simulink model "NEXTCAR_Interface"  (R2017a)
settings: Solver=ode4  StartTime=0.0  StopTime=10000  FixedStep=0.001  RelTol=1e-3  EnableMultiTasking=on
undefined symbols (not defined in the file or in its folder): IO306
libraries: NEXTCAR_Library x50, speedgoatlib_IO106 x4, slrtlib x3, simulink x3, speedgoatlib_fpga_pwm x2, speedgoatlib_IO204 x2, slrttcplib x2, simulink_extras x2, speedgoatlib_fpga x1, xpcseriallib x1, powerlib_meascontrol x1
(part 1 of 2)
settings Model: sg_rtwmakecfg_data=_sglibc_  Creator=G Shaver TC2  LastModifiedBy=joreADM
settings SolverCC: EnableConcurrentExecution=on
settings DataIOCC: SaveFormat=Array  SaveState=on
settings OptimizationCC: BlockReduction=off  OptimizeBlockIOStorage=off  BufferReuse=off  GlobalBufferReuse=off  ExpressionFolding=off  LocalBlockOutputs=off  LifeSpan=inf
settings DebuggingCC: UnderspecifiedInitializationDetection=Classic  MergeDetectMultiDrivingBlocksExec=none  CheckExecutionContextRuntimeOutputMsg=on  SignalResolutionControl=TryResolveAllWithWarning  MultiTaskDSMMsg=warning  MultiTaskCondExecSysMsg=none  SFUnexpectedBacktrackingDiag=warning  SFNoUnconditionalDefaultTransitionDiag=warning
settings HardwareCC: ProdBitPerPointer=32  ProdBitPerSizeT=32  ProdBitPerPtrDiffT=32  ProdLargestAtomicFloat=None  ProdWordSize=32  ProdLongLongMode=on  ProdHWDeviceType=Generic->32-bit x86 compatible
settings RTWCC: SystemTargetFile=slrt.tlc  TemplateMakefile=slrt_default_tmf  Description=Simulink Real-Time  RTWCompilerOptimization=on
settings SimulinkRealTimeCC: xPCisDownloadable=off  xPCisModelTimeout=off  xPCModelTimeoutSecs=30
settings ConfigComp: CovMetricSettings=dw  CovHtmlReporting=on  CovSaveCumulativeToWorkspaceVar=on  CovSaveSingleToWorkspaceVar=on

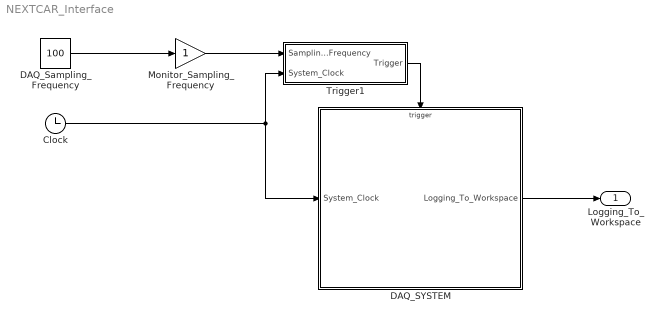
== system NEXTCAR_Interface ==
  Clock : Clock
  DAQ_SYSTEM : Subsystem
  DAQ_Sampling_Frequency : Constant  Value=100
  Monitor_Sampling_Frequency : Gain
  Trigger1 : Subsystem
  Logging_To_Workspace : Outport
  wires:
  Trigger1/1(Trigger) -> DAQ_SYSTEM/Trigger
  DAQ_SYSTEM/1(Logging_To_Workspace) -> Logging_To_Workspace/1
  DAQ_Sampling_Frequency/1 -> Monitor_Sampling_Frequency/1
  Clock/1 -> DAQ_SYSTEM/1(System_Clock), Trigger1/2(System_Clock)
  Monitor_Sampling_Frequency/1 -> Trigger1/1(Sampling_Frequency)

== system NEXTCAR_Interface/DAQ_SYSTEM ==
  note: DEBUG MODE
  System_Clock : Inport
  Trigger1 : TriggerPort  VariantControl=Variant
  Analog_IO_Interface : Subsystem
  Debug_Mode : Constant  Value=0
  Digital_IO_Interface : Subsystem
  Ethernet_Interface : Subsystem  TreatAsAtomicUnit=on
  Logging_Interface : Subsystem
  Mux : Mux
  System_Processing : Subsystem
  Trigger : Subsystem
  Trigger2 : Subsystem
  Logging_To_Workspace : Outport
  tag scope: Debug_Mode=global
  wires:
  Mux/1 -> Logging_Interface/1(Logging_Data), Logging_To_Workspace/1
  Trigger/1(Trigger) -> Ethernet_Interface/Trigger
  Debug_Mode/1 -> [Debug_Mode]
  System_Clock/1 -> Trigger2/1(System_Clock), Trigger/1(System_Clock)
  Trigger2/1(Trigger) -> Logging_Interface/2(Clock_Trigger)
  Analog_IO_Interface/1(Signal_Logging) -> Mux/1
  System_Processing/1(Signal_Logging) -> Mux/4
  Ethernet_Interface/1(Signal_Logging) -> Mux/3
  Digital_IO_Interface/1(Signal_Logging) -> Mux/2

== system NEXTCAR_Interface/Trigger1 ==
  Sampling_Frequency : Inport
  System_Clock : Inport  Port=2
  Constant : Constant
  Divide : Product  Inputs=*/
  Divide1 : Product  Inputs=*/
  Floor : Rounding
  Memory : Memory  InheritSampleTime=on
  Relational Operator : RelationalOperator  Operator=>  OutDataTypeStr=boolean  RndMeth=Simplest
  Trigger : Outport
  wires:
  System_Clock/1 -> Divide/1
  Relational Operator/1 -> Trigger/1
  Divide/1 -> Floor/1
  Memory/1 -> Relational Operator/2
  Floor/1 -> Memory/1, Relational Operator/1
  Sampling_Frequency/1 -> Divide1/2
  Divide1/1 -> Divide/2
  Constant/1 -> Divide1/1

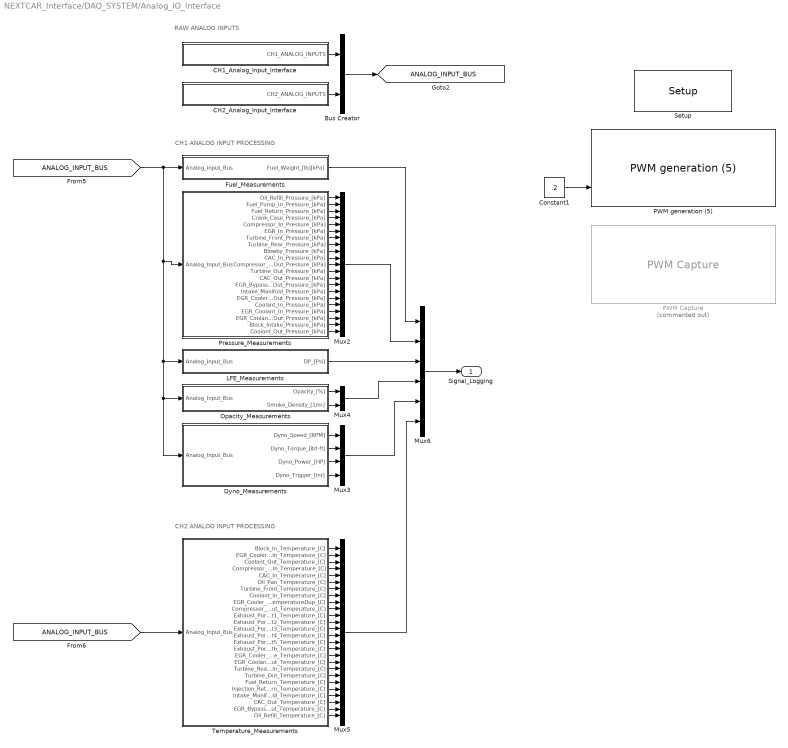
== system NEXTCAR_Interface/DAQ_SYSTEM/Analog_IO_Interface ==
  note: CH2 ANALOG INPUT PROCESSING
  note: CH1 ANALOG INPUT PROCESSING
  note: RAW ANALOG INPUTS
  Bus Creator : BusCreator  Inputs=2
  CH1_Analog_Input_Interface : Subsystem
  CH2_Analog_Input_Interface : Subsystem
  Constant1 : Constant  Value=.2
  Dyno_Measurements : Subsystem
  Fuel_Measurements : Subsystem
  LFE_Measurements : Subsystem
  Mux2 : Mux  Inputs=21
  Mux3 : Mux
  Mux4 : Mux  Inputs=2
  Mux5 : Mux  Inputs=26
  Mux6 : Mux  Inputs=6
  Opacity_Measurements : Subsystem
  PWM Capture : speedgoatlib_fpga_pwm/PWM Capture  Commented=on  id=1  chan=[1]  ts=0.001  pciSlot=-1  board=IO306-25k  captureMode=High transitions triggered  captureTimeout=0  showHighDuration=on  showLowDuration=on  showPeriod=on  showDC16=off  showDC8=off  showTOn=off  showTOff=off  showValidData=off
      settings: SourceProductName=Simulink Real-Time: Speedgoat I/O Driver Library
  PWM generation (5) : speedgoatlib_fpga_pwm/PWM generation (5)  id=1  chan=[1]  board=IO306-25k  ts=-1  pciSlot=-1  symmetric=Symmetric - PWM generation is centered around half the period  b_is_complement_of_a=Independent of PWM A output  deadband=[0.0]  period=0.001  frequency=1000  ticks=32999  a_on=[0]  a_off=[0]  pwm_a_dc=[0.0]  b_on=[0]  b_off=[0]  pwm_b_dc=[0]  c_on=[0.0]  c_off=[0.0]  protection=Disabled: A and B can be high at the same moment  enable_latch_half_period=off  trigger_duration=[1e-6]  trigger_period_start=off  trigger_half_of_the_period=off  trigger_a_on=off  trigger_a_off=off  trigger_b_on=off  trigger_b_off=off  show_a_input=on  show_b_input=on  show_c_input=off  show_period_input=off  show_force_stop_input=off  idle_a=Low when PWM generation is halted  idle_b=Low when PWM generation is halted  idle_c=Low when PWM generation is halted  cancels_pwm_generation=on  invert_a=off  invert_b=off  invert_c=off
      settings: SourceProductName=Simulink Real-Time: Speedgoat I/O Driver Library
  Pressure_Measurements : Subsystem
  Setup : speedgoatlib_fpga/Setup/Setup  board=IO306-25k  id=1  frontIO=None  rearIO=None  bitstreamFile=speedgoat_IO306_25k_CI_01697  timestamp_string=00/00/00 00:00:00  ProgSpiFlash=off  ProgBPIFlash=off  pciSlot=-1  PullRPort0=pull-up 3.3V  VioPort0=3.3V  PullRPort1=pull-up 3.3V  VioPort1=3.3V  PullRPort2=pull-up 3.3V  VioPort2=3.3V  PullRPort3=pull-up 3.3V  VioPort3=3.3V  PullRPort4=pull-up 3.3V  VioPort4=3.3V  PullRPort5=pull-up 3.3V  VioPort5=3.3V  PullRPort6=pull-up 3.3V  VioPort6=3.3V  PullRPort15=pull-up 3.3V  PullRPort31=pull-up 3.3V  PullRPort47=pull-up 3.3V  PullRPort63=pull-up 3.3V
      settings: SourceProductName=Simulink Real-Time: Speedgoat I/O Driver Library
  Temperature_Measurements : Subsystem
  Signal_Logging : Outport
  tag scope: ANALOG_INPUT_BUS=global
  wires:
  Mux6/1 -> Signal_Logging/1
  CH1_Analog_Input_Interface/1(CH1_ANALOG_INPUTS) -> Bus Creator/1
  [ANALOG_INPUT_BUS] -> Dyno_Measurements/1(Analog_Input_Bus), Opacity_Measurements/1(Analog_Input_Bus), LFE_Measurements/1(Analog_Input_Bus), Pressure_Measurements/1(Analog_Input_Bus), Fuel_Measurements/1("Analog_Input_Bus ")
  Dyno_Measurements/1(Dyno_Speed_[RPM]) -> Mux3/1
  Dyno_Measurements/2(Dyno_Torque_[lbf-ft]) -> Mux3/2
  Dyno_Measurements/3(Dyno_Power_[HP]) -> Mux3/3
  Dyno_Measurements/4(Dyno_Trigger_[int]) -> Mux3/4
  Opacity_Measurements/1(Opacity_[%]) -> Mux4/1
  Opacity_Measurements/2(Smoke_Density_[1/m]) -> Mux4/2
  [ANALOG_INPUT_BUS] -> Temperature_Measurements/1(Analog_Input_Bus)
  CH2_Analog_Input_Interface/1(CH2_ANALOG_INPUTS) -> Bus Creator/2
  Bus Creator/1 -> [ANALOG_INPUT_BUS]
  Pressure_Measurements/1(Oil_Refill_Pressure_[kPa]) -> Mux2/1
  Pressure_Measurements/2(Fuel_Pump_In_Pressure_[kPa]) -> Mux2/2
  Pressure_Measurements/3(Fuel_Return_Pressure_[kPa]) -> Mux2/3
  Pressure_Measurements/4(Crank_Case_Pressure_[kPa]) -> Mux2/4
  Pressure_Measurements/5(Compressor_In_Pressure_[kPa]) -> Mux2/5
  Pressure_Measurements/6(EGR_In_Pressure_[kPa]) -> Mux2/6
  Pressure_Measurements/7(Turbine_Front_Pressure_[kPa]) -> Mux2/7
  Pressure_Measurements/8(Turbine_Rear_Pressure_[kPa]) -> Mux2/8
  Pressure_Measurements/9(Blowby_Pressure_[kPa]) -> Mux2/9
  Pressure_Measurements/10(CAC_In_Pressure_[kPa]) -> Mux2/10
  Pressure_Measurements/11(Compressor_Out_Pressure_[kPa]) -> Mux2/11
  Pressure_Measurements/12(Turbine_Out_Pressure_[kPa]) -> Mux2/12
  Pressure_Measurements/13(CAC_Out_Pressure_[kPa]) -> Mux2/13
  Pressure_Measurements/14(EGR_Bypass_Out_Pressure_[kPa]) -> Mux2/14
  Pressure_Measurements/15(Intake_Manifold_Pressure_[kPa]) -> Mux2/15
  Pressure_Measurements/16(EGR_Cooler_Out_Pressure_[kPa]) -> Mux2/16
  Pressure_Measurements/17(Coolant_In_Pressure_[kPa]) -> Mux2/17
  Pressure_Measurements/18(EGR_Coolant_In_Pressure_[kPa]) -> Mux2/18
  Pressure_Measurements/19(EGR_Coolant_Out_Pressure_[kPa]) -> Mux2/19
  Pressure_Measurements/20(Block_Intake_Pressure_[kPa]) -> Mux2/20
  Pressure_Measurements/21(Coolant_Out_Pressure_[kPa]) -> Mux2/21
  Constant1/1 -> PWM generation (5)/2
  Temperature_Measurements/1(Block_In_Temperature_[C]) -> Mux5/1
  Temperature_Measurements/2(EGR_Cooler_In_Temperature_[C]) -> Mux5/2
  Temperature_Measurements/3(Coolant_Out_Temperature_[C]) -> Mux5/3
  Temperature_Measurements/4(Compressor_In_Temperature_[C]) -> Mux5/4
  Temperature_Measurements/5(CAC_In_Temperature_[C]) -> Mux5/5
  Temperature_Measurements/6(Oil_Pan_Temperature_[C]) -> Mux5/6
  Temperature_Measurements/7(Turbine_Front_Temperature_[C]) -> Mux5/7
  Temperature_Measurements/8(Coolant_In_Temperature_[C]) -> Mux5/8
  Temperature_Measurements/9(EGR_Cooler_In_TemperatureDup_[C]) -> Mux5/9
  Temperature_Measurements/10(Compressor_Out_Temperature_[C]) -> Mux5/10
  Temperature_Measurements/11(Exhaust_Port1_Temperature_[C]) -> Mux5/11
  Temperature_Measurements/12(Exhaust_Port2_Temperature_[C]) -> Mux5/12
  Temperature_Measurements/13(Exhaust_Port3_Temperature_[C]) -> Mux5/13
  Temperature_Measurements/14(Exhaust_Port4_Temperature_[C]) -> Mux5/14
  Temperature_Measurements/15(Exhaust_Port5_Temperature_[C]) -> Mux5/15
  Temperature_Measurements/16(Exhaust_Port6_Temperature_[C]) -> Mux5/16
  Temperature_Measurements/17(EGR_Cooler_Intake_Temperature_[C]) -> Mux5/17
  Temperature_Measurements/18(EGR_Coolant_Out_Temperature_[C]) -> Mux5/18
  Temperature_Measurements/19(Turbine_Rear_In_Temperature_[C]) -> Mux5/19
  Temperature_Measurements/20(Turbine_Out_Temperature_[C]) -> Mux5/20
  Temperature_Measurements/21(Fuel_Return_Temperature_[C]) -> Mux5/21
  Temperature_Measurements/22(Injection_Return_Temperature_[C]) -> Mux5/22
  Temperature_Measurements/23(Intake_Manifold_Temperature_[C]) -> Mux5/23
  Temperature_Measurements/24(CAC_Out_Temperature_[C]) -> Mux5/24
  Temperature_Measurements/25(EGR_Bypass_Out_Temperature_[C]) -> Mux5/25
  Temperature_Measurements/26(Oil_Refill_Temperature_[C]) -> Mux5/26
  Fuel_Measurements/1(Fuel_Weight_[lb][kPa]) -> Mux6/1
  Mux2/1 -> Mux6/2
  LFE_Measurements/1(DP_[Psi]) -> Mux6/3
  Mux4/1 -> Mux6/4
  Mux3/1 -> Mux6/5
  Mux5/1 -> Mux6/6

== system NEXTCAR_Interface/DAQ_SYSTEM/Digital_IO_Interface ==
  note: COMMANDED DIGITAL OUTPUTS
  Digital_Output_Interface : Subsystem
  Signal_Logging : Outport
  wires:
  Digital_Output_Interface/1(Signal_Logging) -> Signal_Logging/1

== system NEXTCAR_Interface/DAQ_SYSTEM/Ethernet_Interface ==
  Trigger : TriggerPort  VariantControl=Variant
  ASCII_Encode : xpcseriallib/ASCII Encode   format=%d  nvars=1  maxlength=3  vartypes={ 'double' }
      settings: SourceProductName=Simulink Real-Time  SourceProductBaseCode=XP
  Constant : Constant  Value=100
  Constant1 : Constant
  Mux : Mux  Inputs=2
  TCP_Client_Configure : slrttcplib/TCP Client Configure  Priority=-1  useHostTargetConn=off  clientAddress=192.168.7.2  clientPort=65001  SubnetMask=255.255.255.2  Gateway=0.0.0.0  remoteAddress=192.168.7.222  remotePort=10006  PciBus=7  PciSlot=6
      settings: SourceProductName=Simulink Real-Time  SourceProductBaseCode=XP
  TCP_Send : slrttcplib/TCP Send  socketAddPortVal=Client: 192.168.7.2:65001  sampleTime=-1
      settings: SourceProductName=Simulink Real-Time  SourceProductBaseCode=XP
  Width1 : Width
  Signal_Logging : Outport
  wires:
  Constant/1 -> ASCII_Encode/1
  Width1/1 -> TCP_Send/3
  ASCII_Encode/1 -> TCP_Send/2, Width1/1
  Constant1/1 -> TCP_Send/1, TCP_Client_Configure/1
  TCP_Client_Configure/1 -> Mux/1  "TCP_Client_Configure_Status_[-]"
  TCP_Send/1 -> Mux/2  "TCP_Send_Status_[-]"
  Mux/1 -> Signal_Logging/1

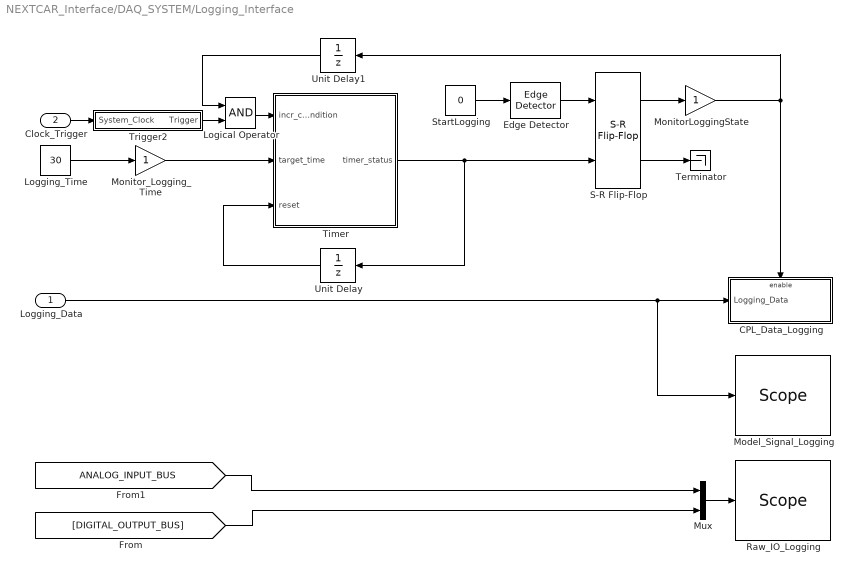
== system NEXTCAR_Interface/DAQ_SYSTEM/Logging_Interface ==
  Logging_Data : Inport
  Clock_Trigger : Inport  Port=2
  CPL_Data_Logging : Subsystem  TreatAsAtomicUnit=on
  Edge Detector : powerlib_meascontrol/Logic/Edge Detector  model=Either  ic=0  Ts=-1
      settings: SourceProductName=Simscape Power Systems  SourceProductBaseCode=PS
  Logging_Time : Constant  Value=30
  Logical Operator : Logic  AllPortsSameDT=off  OutDataTypeStr=boolean
  "Model_Signal_Logging " : slrtlib/Displays and Logging/Scope   scopeno=1  scopetype=File  autostart=on  viewmode=Graphical redraw  formatstr='%15.6f'  grid=on  ylimits=[0,0]  nosamples=250  noprepostsamples=0  interleave=1  triggermode=FreeRun  triggersignal=1  trigsignalfromport=on  triggerlevel=0.5  triggerslope=Rising  triggerscope=1  triggersample=0  filename=ModelLog.dat  mode=Lazy  writesize=512  autorestart=on  dynamicfilemode=off  maxwritefilesize=512*11718750
  MonitorLoggingState : Gain
  Monitor_Logging_Time : Gain
  Mux : Mux  Inputs=2
  Raw_IO_Logging : slrtlib/Displays and Logging/Scope   scopeno=2  scopetype=File  autostart=on  viewmode=Graphical redraw  formatstr='%15.6f'  grid=on  ylimits=[0,0]  nosamples=250  noprepostsamples=0  interleave=1  triggermode=FreeRun  triggersignal=1  trigsignalfromport=on  triggerlevel=0.5  triggerslope=Rising  triggerscope=1  triggersample=0  filename=RawIOLog.dat  mode=Lazy  writesize=512  autorestart=on  dynamicfilemode=off  maxwritefilesize=512*11718750
  S-R Flip-Flop : simulink_extras/Flip Flops/S-R Flip-Flop  initial_condition=0
  StartLogging : Constant  Value=0
  Terminator : Terminator
  Timer : Subsystem
  Trigger2 : Subsystem
  Unit Delay : UnitDelay  SampleTime=-1
  Unit Delay1 : UnitDelay  SampleTime=-1
  wires:
  S-R Flip-Flop/2 -> Terminator/1
  Edge Detector/1 -> S-R Flip-Flop/1
  StartLogging/1 -> Edge Detector/1
  Timer/1(timer_status) -> Unit Delay/1, S-R Flip-Flop/2
  MonitorLoggingState/1 -> Unit Delay1/1, CPL_Data_Logging/Enable
  Logging_Time/1 -> Monitor_Logging_Time/1
  Clock_Trigger/1 -> Trigger2/1(System_Clock)
  Logging_Data/1 -> "Model_Signal_Logging "/1, CPL_Data_Logging/1(Logging_Data)
  Unit Delay/1 -> Timer/3(reset)
  Monitor_Logging_Time/1 -> Timer/2(target_time)
  S-R Flip-Flop/1 -> MonitorLoggingState/1
  Logical Operator/1 -> Timer/1(incr_condition)
  Trigger2/1(Trigger) -> Logical Operator/2
  Unit Delay1/1 -> Logical Operator/1
  Mux/1 -> Raw_IO_Logging/1
  [DIGITAL_OUTPUT_BUS] -> Mux/2
  [ANALOG_INPUT_BUS] -> Mux/1

== system NEXTCAR_Interface/DAQ_SYSTEM/System_Processing ==
  note: ENGINE SYSTEM CALCULATIONS
  note: ENGINE SYSTEM CONTROLS
  Fuel_System_Control : Subsystem
  Mux1 : Mux  Inputs=2
  Mux2 : Mux  Inputs=2
  Mux4 : Mux  Inputs=2
  Psychrometric_Calculations : Subsystem
  Signal_Logging : Outport
  wires:
  Psychrometric_Calculations/1(LFE_Wet_[kgpm]) -> Mux4/1
  Psychrometric_Calculations/2(LFE_Dry_[kgpm]) -> Mux4/2
  Fuel_System_Control/1(Fuel_Weight_[lb]) -> Mux1/1
  Fuel_System_Control/2(Fuel_Refill_[bool]) -> Mux1/2
  Mux2/1 -> Signal_Logging/1
  Mux4/1 -> Mux2/1
  Mux1/1 -> Mux2/2

== system NEXTCAR_Interface/DAQ_SYSTEM/Trigger ==
  System_Clock : Inport
  Constant : Constant  Value=10
  Divide : Product  Inputs=*/
  Floor : Rounding
  Memory : Memory  InheritSampleTime=on
  Relational Operator : RelationalOperator  Operator=>  OutDataTypeStr=boolean  RndMeth=Simplest
  Trigger : Outport
  wires:
  Floor/1 -> Relational Operator/1, Memory/1
  Constant/1 -> Divide/2
  Memory/1 -> Relational Operator/2
  Divide/1 -> Floor/1
  Relational Operator/1 -> Trigger/1
  System_Clock/1 -> Divide/1

== system NEXTCAR_Interface/DAQ_SYSTEM/Trigger2 ==
  System_Clock : Inport
  Constant : Constant
  Divide : Product  Inputs=*/
  Floor : Rounding
  Memory : Memory  InheritSampleTime=on
  Relational Operator : RelationalOperator  Operator=>  OutDataTypeStr=boolean  RndMeth=Simplest
  Trigger : Outport
  wires:
  System_Clock/1 -> Divide/1
  Relational Operator/1 -> Trigger/1
  Divide/1 -> Floor/1
  Memory/1 -> Relational Operator/2
  Constant/1 -> Divide/2
  Floor/1 -> Memory/1, Relational Operator/1

== system NEXTCAR_Interface/DAQ_SYSTEM/Analog_IO_Interface/CH1_Analog_Input_Interface ==
  Analog input : speedgoatlib_IO106/Analog input  id=1  channels=64  range=1  coupling=1  ts=-1  initiator=1  pciSlot=[7,4]
      settings: SourceProductName=Simulink Real-Time: Speedgoat I/O Driver Library
  Bus Creator : BusCreator  Inputs=64
  Demux : Demux  Outputs=64
  Setup : speedgoatlib_IO106/Setup  group=Module setup  id=1  cal=on  initiator=Initiator  pciSlot=[7,4]  adChannel=64  adRange=+-10V  adCoupling=Single-ended
      settings: SourceProductName=Simulink Real-Time: Speedgoat I/O Driver Library
  CH1_ANALOG_INPUTS : Outport
  wires:
  Analog input/1 -> Demux/1
  Demux/27 -> Bus Creator/27  "CH1_ANALOG_INPUT_27"
  Demux/18 -> Bus Creator/18  "CH1_ANALOG_INPUT_18"
  Demux/5 -> Bus Creator/5  "CH1_ANALOG_INPUT_5"
  Demux/28 -> Bus Creator/28  "CH1_ANALOG_INPUT_28"
  Demux/14 -> Bus Creator/14  "CH1_ANALOG_INPUT_14"
  Demux/29 -> Bus Creator/29  "CH1_ANALOG_INPUT_29"
  Demux/16 -> Bus Creator/16  "CH1_ANALOG_INPUT_16"
  Demux/21 -> Bus Creator/21  "CH1_ANALOG_INPUT_21"
  Demux/24 -> Bus Creator/24  "CH1_ANALOG_INPUT_24"
  Demux/15 -> Bus Creator/15  "CH1_ANALOG_INPUT_15"
  Demux/31 -> Bus Creator/31  "CH1_ANALOG_INPUT_31"
  Demux/32 -> Bus Creator/32  "CH1_ANALOG_INPUT_32"
  Demux/33 -> Bus Creator/33  "CH1_ANALOG_INPUT_33"
  Demux/30 -> Bus Creator/30  "CH1_ANALOG_INPUT_30"
  Demux/2 -> Bus Creator/2  "CH1_ANALOG_INPUT_2"
  Demux/22 -> Bus Creator/22  "CH1_ANALOG_INPUT_22"
  Demux/4 -> Bus Creator/4  "CH1_ANALOG_INPUT_4"
  Demux/19 -> Bus Creator/19  "CH1_ANALOG_INPUT_19"
  Demux/6 -> Bus Creator/6  "CH1_ANALOG_INPUT_6"
  Demux/25 -> Bus Creator/25  "CH1_ANALOG_INPUT_25"
  Demux/13 -> Bus Creator/13  "CH1_ANALOG_INPUT_13"
  Demux/23 -> Bus Creator/23  "CH1_ANALOG_INPUT_23"
  Demux/34 -> Bus Creator/34  "CH1_ANALOG_INPUT_34"
  Demux/1 -> Bus Creator/1  "CH1_ANALOG_INPUT_1"
  Demux/7 -> Bus Creator/7  "CH1_ANALOG_INPUT_7"
  Demux/8 -> Bus Creator/8  "CH1_ANALOG_INPUT_8"
  Demux/3 -> Bus Creator/3  "CH1_ANALOG_INPUT_3"
  Demux/11 -> Bus Creator/11  "CH1_ANALOG_INPUT_11"
  Demux/10 -> Bus Creator/10  "CH1_ANALOG_INPUT_10"
  Demux/12 -> Bus Creator/12  "CH1_ANALOG_INPUT_12"
  Demux/9 -> Bus Creator/9  "CH1_ANALOG_INPUT_9"
  Demux/17 -> Bus Creator/17  "CH1_ANALOG_INPUT_17"
  Demux/20 -> Bus Creator/20  "CH1_ANALOG_INPUT_20"
  Demux/26 -> Bus Creator/26  "CH1_ANALOG_INPUT_26"
  Demux/50 -> Bus Creator/50  "CH1_ANALOG_INPUT_50"
  Demux/52 -> Bus Creator/52  "CH1_ANALOG_INPUT_52"
  Demux/53 -> Bus Creator/53  "CH1_ANALOG_INPUT_53"
  Demux/54 -> Bus Creator/54  "CH1_ANALOG_INPUT_54"
  Demux/59 -> Bus Creator/59  "CH1_ANALOG_INPUT_59"
  Demux/60 -> Bus Creator/60  "CH1_ANALOG_INPUT_60"
  Demux/46 -> Bus Creator/46  "CH1_ANALOG_INPUT_46"
  Demux/57 -> Bus Creator/57  "CH1_ANALOG_INPUT_57"
  Demux/37 -> Bus Creator/37  "CH1_ANALOG_INPUT_37"
  Demux/41 -> Bus Creator/41  "CH1_ANALOG_INPUT_41"
  Demux/49 -> Bus Creator/49  "CH1_ANALOG_INPUT_49"
  Demux/58 -> Bus Creator/58  "CH1_ANALOG_INPUT_58"
  Demux/56 -> Bus Creator/56  "CH1_ANALOG_INPUT_56"
  Demux/44 -> Bus Creator/44  "CH1_ANALOG_INPUT_44"
  Demux/61 -> Bus Creator/61  "CH1_ANALOG_INPUT_61"
  Demux/62 -> Bus Creator/62  "CH1_ANALOG_INPUT_62"
  Demux/63 -> Bus Creator/63  "CH1_ANALOG_INPUT_63"
  Demux/55 -> Bus Creator/55  "CH1_ANALOG_INPUT_55"
  Demux/64 -> Bus Creator/64  "CH1_ANALOG_INPUT_64"
  Demux/39 -> Bus Creator/39  "CH1_ANALOG_INPUT_39"
  Demux/47 -> Bus Creator/47  "CH1_ANALOG_INPUT_47"
  Demux/40 -> Bus Creator/40  "CH1_ANALOG_INPUT_40"
  Demux/51 -> Bus Creator/51  "CH1_ANALOG_INPUT_51"
  Demux/45 -> Bus Creator/45  "CH1_ANALOG_INPUT_45"
  Demux/36 -> Bus Creator/36  "CH1_ANALOG_INPUT_36"
  Demux/38 -> Bus Creator/38  "CH1_ANALOG_INPUT_38"
  Demux/42 -> Bus Creator/42  "CH1_ANALOG_INPUT_42"
  Demux/48 -> Bus Creator/48  "CH1_ANALOG_INPUT_48"
  Demux/35 -> Bus Creator/35  "CH1_ANALOG_INPUT_35"
  Demux/43 -> Bus Creator/43  "CH1_ANALOG_INPUT_43"
  Bus Creator/1 -> CH1_ANALOG_INPUTS/1  "CH1_ANALOG_INPUTS"

== system NEXTCAR_Interface/DAQ_SYSTEM/Analog_IO_Interface/CH2_Analog_Input_Interface ==
  Analog input : speedgoatlib_IO106/Analog input  id=2  channels=64  range=1  coupling=1  ts=-1  initiator=1  pciSlot=[7,5]
      settings: SourceProductName=Simulink Real-Time: Speedgoat I/O Driver Library
  Bus Creator : BusCreator  Inputs=64
  Demux : Demux  Outputs=64
  Setup : speedgoatlib_IO106/Setup  group=Module setup  id=2  cal=on  initiator=Initiator  pciSlot=[7,5]  adChannel=64  adRange=+-10V  adCoupling=Single-ended
      settings: SourceProductName=Simulink Real-Time: Speedgoat I/O Driver Library
  CH2_ANALOG_INPUTS : Outport
  wires:
  Bus Creator/1 -> CH2_ANALOG_INPUTS/1  "CH2_ANALOG_INPUTS"
  Demux/43 -> Bus Creator/43  "CH2_ANALOG_INPUT_43"
  Demux/35 -> Bus Creator/35  "CH2_ANALOG_INPUT_35"
  Demux/48 -> Bus Creator/48  "CH2_ANALOG_INPUT_48"
  Demux/42 -> Bus Creator/42  "CH2_ANALOG_INPUT_42"
  Demux/38 -> Bus Creator/38  "CH2_ANALOG_INPUT_38"
  Demux/36 -> Bus Creator/36  "CH2_ANALOG_INPUT_36"
  Demux/45 -> Bus Creator/45  "CH2_ANALOG_INPUT_45"
  Demux/51 -> Bus Creator/51  "CH2_ANALOG_INPUT_51"
  Demux/40 -> Bus Creator/40  "CH2_ANALOG_INPUT_40"
  Demux/47 -> Bus Creator/47  "CH2_ANALOG_INPUT_47"
  Demux/39 -> Bus Creator/39  "CH2_ANALOG_INPUT_39"
  Demux/64 -> Bus Creator/64  "CH2_ANALOG_INPUT_64"
  Demux/55 -> Bus Creator/55  "CH2_ANALOG_INPUT_55"
  Demux/63 -> Bus Creator/63  "CH2_ANALOG_INPUT_63"
  Demux/62 -> Bus Creator/62  "CH2_ANALOG_INPUT_62"
  Demux/61 -> Bus Creator/61  "CH2_ANALOG_INPUT_61"
  Demux/44 -> Bus Creator/44  "CH2_ANALOG_INPUT_44"
  Demux/56 -> Bus Creator/56  "CH2_ANALOG_INPUT_56"
  Demux/58 -> Bus Creator/58  "CH2_ANALOG_INPUT_58"
  Demux/49 -> Bus Creator/49  "CH2_ANALOG_INPUT_49"
  Demux/41 -> Bus Creator/41  "CH2_ANALOG_INPUT_41"
  Demux/37 -> Bus Creator/37  "CH2_ANALOG_INPUT_37"
  Demux/57 -> Bus Creator/57  "CH2_ANALOG_INPUT_57"
  Demux/46 -> Bus Creator/46  "CH2_ANALOG_INPUT_46"
  Demux/60 -> Bus Creator/60  "CH2_ANALOG_INPUT_60"
  Demux/59 -> Bus Creator/59  "CH2_ANALOG_INPUT_59"
  Demux/54 -> Bus Creator/54  "CH2_ANALOG_INPUT_54"
  Demux/53 -> Bus Creator/53  "CH2_ANALOG_INPUT_53"
  Demux/52 -> Bus Creator/52  "CH2_ANALOG_INPUT_52"
  Demux/50 -> Bus Creator/50  "CH2_ANALOG_INPUT_50"
  Demux/26 -> Bus Creator/26  "CH2_ANALOG_INPUT_26"
  Demux/20 -> Bus Creator/20  "CH2_ANALOG_INPUT_20"
  Demux/17 -> Bus Creator/17  "CH2_ANALOG_INPUT_17"
  Demux/9 -> Bus Creator/9  "CH2_ANALOG_INPUT_9"
  Demux/12 -> Bus Creator/12  "CH2_ANALOG_INPUT_12"
  Demux/10 -> Bus Creator/10  "CH2_ANALOG_INPUT_10"
  Demux/11 -> Bus Creator/11  "CH2_ANALOG_INPUT_11"
  Demux/3 -> Bus Creator/3  "CH2_ANALOG_INPUT_3"
  Demux/8 -> Bus Creator/8  "CH2_ANALOG_INPUT_8"
  Demux/7 -> Bus Creator/7  "CH2_ANALOG_INPUT_7"
  Demux/1 -> Bus Creator/1  "CH2_ANALOG_INPUT_1"
  Demux/34 -> Bus Creator/34  "CH2_ANALOG_INPUT_34"
  Demux/23 -> Bus Creator/23  "CH2_ANALOG_INPUT_23"
  Demux/13 -> Bus Creator/13  "CH2_ANALOG_INPUT_13"
  Demux/25 -> Bus Creator/25  "CH2_ANALOG_INPUT_25"
  Demux/6 -> Bus Creator/6  "CH2_ANALOG_INPUT_6"
  Demux/19 -> Bus Creator/19  "CH2_ANALOG_INPUT_19"
  Demux/4 -> Bus Creator/4  "CH2_ANALOG_INPUT_4"
  Demux/22 -> Bus Creator/22  "CH2_ANALOG_INPUT_22"
  Demux/2 -> Bus Creator/2  "CH2_ANALOG_INPUT_2"
  Demux/30 -> Bus Creator/30  "CH2_ANALOG_INPUT_30"
  Demux/33 -> Bus Creator/33  "CH2_ANALOG_INPUT_33"
  Demux/32 -> Bus Creator/32  "CH2_ANALOG_INPUT_32"
  Demux/31 -> Bus Creator/31  "CH2_ANALOG_INPUT_31"
  Demux/15 -> Bus Creator/15  "CH2_ANALOG_INPUT_15"
  Demux/24 -> Bus Creator/24  "CH2_ANALOG_INPUT_24"
  Demux/21 -> Bus Creator/21  "CH2_ANALOG_INPUT_21"
  Demux/16 -> Bus Creator/16  "CH2_ANALOG_INPUT_16"
  Demux/29 -> Bus Creator/29  "CH2_ANALOG_INPUT_29"
  Demux/14 -> Bus Creator/14  "CH2_ANALOG_INPUT_14"
  Demux/28 -> Bus Creator/28  "CH2_ANALOG_INPUT_28"
  Demux/5 -> Bus Creator/5  "CH2_ANALOG_INPUT_5"
  Demux/18 -> Bus Creator/18  "CH2_ANALOG_INPUT_18"
  Demux/27 -> Bus Creator/27  "CH2_ANALOG_INPUT_27"
  Analog input/1 -> Demux/1

== system NEXTCAR_Interface/DAQ_SYSTEM/Analog_IO_Interface/Dyno_Measurements ==
  Analog_Input_Bus : Inport
  Bus Selector1 : BusSelector  OutputSignals=CH1_ANALOG_INPUTS.CH1_ANALOG_INPUT_34
  Bus Selector2 : BusSelector  OutputSignals=CH1_ANALOG_INPUTS.CH1_ANALOG_INPUT_35
  Bus Selector3 : BusSelector  OutputSignals=CH1_ANALOG_INPUTS.CH1_ANALOG_INPUT_36
  Bus Selector5 : BusSelector  OutputSignals=CH1_ANALOG_INPUTS.CH1_ANALOG_INPUT_33
  ConvertAnalogToDyno : NEXTCAR_Library/ConvertAnalogToDyno  speed_max=4200  torque_max=2500  power_max=67  trigger_max=67
      settings: SourceProductName=NEXTCAR Library
  Monitor_Dyno_Power_[HP] : Gain
  Monitor_Dyno_Speed_[RPM] : Gain
  Monitor_Dyno_Torque_[lbf-ft] : Gain
  Monitor_Dyno_Trigger_[int] : Gain
  Dyno_Speed_[RPM] : Outport
  Dyno_Torque_[lbf-ft] : Outport  Port=2
  Dyno_Power_[HP] : Outport  Port=3
  Dyno_Trigger_[int] : Outport  Port=4
  wires:
  Bus Selector5/1 -> ConvertAnalogToDyno/1  "<CH1_ANALOG_INPUT_33>"
  ConvertAnalogToDyno/1 -> Monitor_Dyno_Speed_[RPM]/1
  Monitor_Dyno_Speed_[RPM]/1 -> Dyno_Speed_[RPM]/1
  ConvertAnalogToDyno/2 -> Monitor_Dyno_Torque_[lbf-ft]/1
  Bus Selector1/1 -> ConvertAnalogToDyno/2  "<CH1_ANALOG_INPUT_34>"
  Monitor_Dyno_Torque_[lbf-ft]/1 -> Dyno_Torque_[lbf-ft]/1
  Bus Selector2/1 -> ConvertAnalogToDyno/3  "<CH1_ANALOG_INPUT_35>"
  ConvertAnalogToDyno/3 -> Monitor_Dyno_Power_[HP]/1
  Monitor_Dyno_Power_[HP]/1 -> Dyno_Power_[HP]/1
  Monitor_Dyno_Trigger_[int]/1 -> Dyno_Trigger_[int]/1
  Bus Selector3/1 -> ConvertAnalogToDyno/4  "<CH1_ANALOG_INPUT_36>"
  Analog_Input_Bus/1 -> Bus Selector3/1, Bus Selector2/1, Bus Selector1/1, Bus Selector5/1
  ConvertAnalogToDyno/4 -> Monitor_Dyno_Trigger_[int]/1

== system NEXTCAR_Interface/DAQ_SYSTEM/Analog_IO_Interface/Fuel_Measurements ==
  "Analog_Input_Bus " : Inport
  Bus Selector : BusSelector  OutputSignals=CH1_ANALOG_INPUTS.CH1_ANALOG_INPUT_1
  Fuel_Weight : Subsystem
  Monitor_Fuel_Weight_[lb] : Gain
  Fuel_Weight_[lb][kPa] : Outport
  wires:
  Bus Selector/1 -> Fuel_Weight/1(Voltage)  "<CH1_ANALOG_INPUT_1>"
  "Analog_Input_Bus "/1 -> Bus Selector/1
  Fuel_Weight/1(Weight) -> Monitor_Fuel_Weight_[lb]/1
  Monitor_Fuel_Weight_[lb]/1 -> Fuel_Weight_[lb][kPa]/1, [Fuel_Weight]

== system NEXTCAR_Interface/DAQ_SYSTEM/Analog_IO_Interface/LFE_Measurements ==
  Analog_Input_Bus : Inport
  Bus Selector : BusSelector  OutputSignals=CH1_ANALOG_INPUTS.CH1_ANALOG_INPUT_27
  LFE_Linear_Sensor_Calibration : Subsystem  mask{slope=.0361, offset=0}
      mask prompts: slope "What is the calibration slope (in units/volt)?"; offset "What is the calibration offeset (in units)?"
      mask init:
      | str1 = ['slope = ' num2str(slope)];
      | str2 = ['offset = ' num2str(offset)];
      mask Display:
      | text(0.5, 2/3, str1, 'horizontalAlignment', 'center','verticalAlignment', 'middle')
      | text(0.5, 1/3, str2, 'horizontalAlignment', 'center', 'verticalAlignment', 'middle')
  Monitor_DP_[Psi] : Gain
  DP_[Psi] : Outport
  tag scope: DP=global
  wires:
  Analog_Input_Bus/1 -> Bus Selector/1
  LFE_Linear_Sensor_Calibration/1(Out1) -> Monitor_DP_[Psi]/1
  Bus Selector/1 -> LFE_Linear_Sensor_Calibration/1(In1)  "<CH1_ANALOG_INPUT_27>"
  Monitor_DP_[Psi]/1 -> [DP], DP_[Psi]/1

== system NEXTCAR_Interface/DAQ_SYSTEM/Analog_IO_Interface/Opacity_Measurements ==
  Analog_Input_Bus : Inport
  Bus Selector1 : BusSelector  OutputSignals=CH1_ANALOG_INPUTS.CH1_ANALOG_INPUT_30
  Bus Selector5 : BusSelector  OutputSignals=CH1_ANALOG_INPUTS.CH1_ANALOG_INPUT_29
  ConvertAnalogToPercent1 : NEXTCAR_Library/ConvertAnalogToPercent  V_Max=10
      settings: SourceProductName=NEXTCAR Library
  ConvertAnalogToPercent2 : NEXTCAR_Library/ConvertAnalogToPercent  V_Max=10
      settings: SourceProductName=NEXTCAR Library
  Monitor_Opacity_[%] : Gain
  Monitor_Smoke_Density_[1/m] : Gain
  Opacity_[%] : Outport
  Smoke_Density_[1/m] : Outport  Port=2
  wires:
  ConvertAnalogToPercent2/1 -> Monitor_Opacity_[%]/1
  Analog_Input_Bus/1 -> Bus Selector1/1, Bus Selector5/1
  Bus Selector5/1 -> ConvertAnalogToPercent2/1  "<CH1_ANALOG_INPUT_29>"
  Monitor_Opacity_[%]/1 -> Opacity_[%]/1
  Monitor_Smoke_Density_[1/m]/1 -> Smoke_Density_[1/m]/1
  ConvertAnalogToPercent1/1 -> Monitor_Smoke_Density_[1/m]/1
  Bus Selector1/1 -> ConvertAnalogToPercent1/1  "<CH1_ANALOG_INPUT_30>"

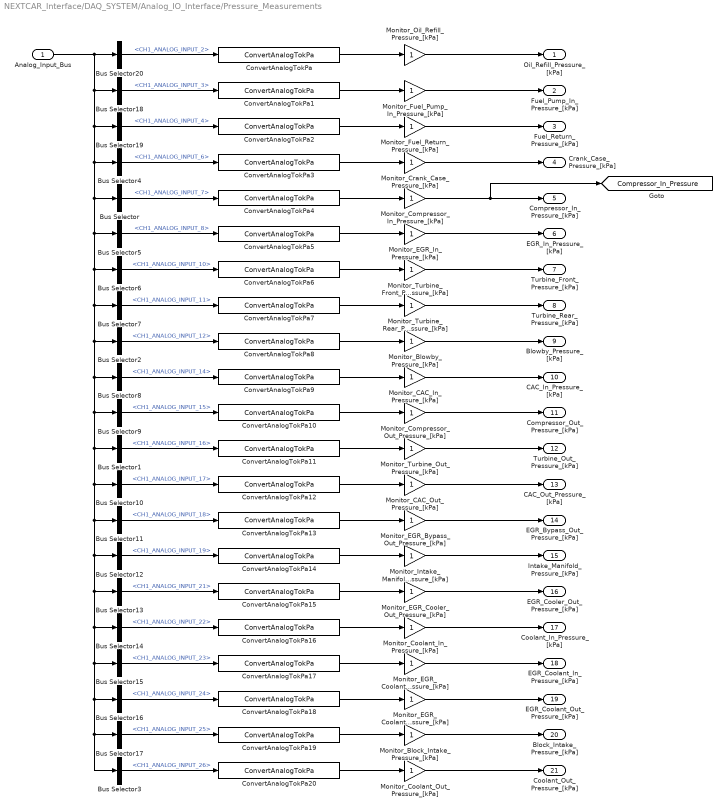
== system NEXTCAR_Interface/DAQ_SYSTEM/Analog_IO_Interface/Pressure_Measurements ==
  Analog_Input_Bus : Inport
  Bus Selector : BusSelector  OutputSignals=CH1_ANALOG_INPUTS.CH1_ANALOG_INPUT_7
  Bus Selector1 : BusSelector  OutputSignals=CH1_ANALOG_INPUTS.CH1_ANALOG_INPUT_16
  Bus Selector10 : BusSelector  OutputSignals=CH1_ANALOG_INPUTS.CH1_ANALOG_INPUT_17
  Bus Selector11 : BusSelector  OutputSignals=CH1_ANALOG_INPUTS.CH1_ANALOG_INPUT_18
  Bus Selector12 : BusSelector  OutputSignals=CH1_ANALOG_INPUTS.CH1_ANALOG_INPUT_19
  Bus Selector13 : BusSelector  OutputSignals=CH1_ANALOG_INPUTS.CH1_ANALOG_INPUT_21
  Bus Selector14 : BusSelector  OutputSignals=CH1_ANALOG_INPUTS.CH1_ANALOG_INPUT_22
  Bus Selector15 : BusSelector  OutputSignals=CH1_ANALOG_INPUTS.CH1_ANALOG_INPUT_23
  Bus Selector16 : BusSelector  OutputSignals=CH1_ANALOG_INPUTS.CH1_ANALOG_INPUT_24
  Bus Selector17 : BusSelector  OutputSignals=CH1_ANALOG_INPUTS.CH1_ANALOG_INPUT_25
  Bus Selector18 : BusSelector  OutputSignals=CH1_ANALOG_INPUTS.CH1_ANALOG_INPUT_3
  Bus Selector19 : BusSelector  OutputSignals=CH1_ANALOG_INPUTS.CH1_ANALOG_INPUT_4
  Bus Selector2 : BusSelector  OutputSignals=CH1_ANALOG_INPUTS.CH1_ANALOG_INPUT_12
  Bus Selector20 : BusSelector  OutputSignals=CH1_ANALOG_INPUTS.CH1_ANALOG_INPUT_2
  Bus Selector3 : BusSelector  OutputSignals=CH1_ANALOG_INPUTS.CH1_ANALOG_INPUT_26
  Bus Selector4 : BusSelector  OutputSignals=CH1_ANALOG_INPUTS.CH1_ANALOG_INPUT_6
  Bus Selector5 : BusSelector  OutputSignals=CH1_ANALOG_INPUTS.CH1_ANALOG_INPUT_8
  Bus Selector6 : BusSelector  OutputSignals=CH1_ANALOG_INPUTS.CH1_ANALOG_INPUT_10
  Bus Selector7 : BusSelector  OutputSignals=CH1_ANALOG_INPUTS.CH1_ANALOG_INPUT_11
  Bus Selector8 : BusSelector  OutputSignals=CH1_ANALOG_INPUTS.CH1_ANALOG_INPUT_14
  Bus Selector9 : BusSelector  OutputSignals=CH1_ANALOG_INPUTS.CH1_ANALOG_INPUT_15
  ConvertAnalogTokPa : NEXTCAR_Library/ConvertAnalogTokPa  P_Max=8
      settings: SourceProductName=NEXTCAR Library
  ConvertAnalogTokPa{1..2,5..7,10..20} (16 alike) : NEXTCAR_Library/ConvertAnalogTokPa  P_Max=5
      settings: SourceProductName=NEXTCAR Library
  ConvertAnalogTokPa{3..4,8..9} (4 alike) : NEXTCAR_Library/ConvertAnalogTokPa  P_Max=2
      settings: SourceProductName=NEXTCAR Library
  Monitor_Block_Intake_Pressure_[kPa] : Gain
  Monitor_Blowby_Pressure_[kPa] : Gain
  Monitor_CAC_In_Pressure_[kPa] : Gain
  Monitor_CAC_Out_Pressure_[kPa] : Gain
  Monitor_Compressor_In_Pressure_[kPa] : Gain
  Monitor_Compressor_Out_Pressure_[kPa] : Gain
  Monitor_Coolant_In_Pressure_[kPa] : Gain
  Monitor_Coolant_Out_Pressure_[kPa] : Gain
  Monitor_Crank_Case_Pressure_[kPa] : Gain
  Monitor_EGR_Bypass_Out_Pressure_[kPa] : Gain
  Monitor_EGR_Coolant_In_Pressure_[kPa] : Gain
  Monitor_EGR_Coolant_Out_Pressure_[kPa] : Gain
  Monitor_EGR_Cooler_Out_Pressure_[kPa] : Gain
  Monitor_EGR_In_Pressure_[kPa] : Gain
  Monitor_Fuel_Pump_In_Pressure_[kPa] : Gain
  Monitor_Fuel_Return_Pressure_[kPa] : Gain
  Monitor_Intake_Manifold_Pressure_[kPa] : Gain
  Monitor_Oil_Refill_Pressure_[kPa] : Gain
  Monitor_Turbine_Front_Pressure_[kPa] : Gain
  Monitor_Turbine_Out_Pressure_[kPa] : Gain
  Monitor_Turbine_Rear_Pressure_[kPa] : Gain
  Oil_Refill_Pressure_[kPa] : Outport
  Fuel_Pump_In_Pressure_[kPa] : Outport  Port=2
  Fuel_Return_Pressure_[kPa] : Outport  Port=3
  Crank_Case_Pressure_[kPa] : Outport  Port=4
  Compressor_In_Pressure_[kPa] : Outport  Port=5
  EGR_In_Pressure_[kPa] : Outport  Port=6
  Turbine_Front_Pressure_[kPa] : Outport  Port=7
  Turbine_Rear_Pressure_[kPa] : Outport  Port=8
  Blowby_Pressure_[kPa] : Outport  Port=9
  CAC_In_Pressure_[kPa] : Outport  Port=10
  Compressor_Out_Pressure_[kPa] : Outport  Port=11
  Turbine_Out_Pressure_[kPa] : Outport  Port=12
  CAC_Out_Pressure_[kPa] : Outport  Port=13
  EGR_Bypass_Out_Pressure_[kPa] : Outport  Port=14
  Intake_Manifold_Pressure_[kPa] : Outport  Port=15
  EGR_Cooler_Out_Pressure_[kPa] : Outport  Port=16
  Coolant_In_Pressure_[kPa] : Outport  Port=17
  EGR_Coolant_In_Pressure_[kPa] : Outport  Port=18
  EGR_Coolant_Out_Pressure_[kPa] : Outport  Port=19
  Block_Intake_Pressure_[kPa] : Outport  Port=20
  Coolant_Out_Pressure_[kPa] : Outport  Port=21
  tag scope: Compressor_In_Pressure=global
  wires:
  Bus Selector/1 -> ConvertAnalogTokPa4/1  "<CH1_ANALOG_INPUT_7>"
  Bus Selector1/1 -> ConvertAnalogTokPa11/1  "<CH1_ANALOG_INPUT_16>"
  Monitor_Compressor_In_Pressure_[kPa]/1 -> [Compressor_In_Pressure], Compressor_In_Pressure_[kPa]/1
  Monitor_Turbine_Out_Pressure_[kPa]/1 -> Turbine_Out_Pressure_[kPa]/1
  Bus Selector3/1 -> ConvertAnalogTokPa20/1  "<CH1_ANALOG_INPUT_26>"
  Monitor_Coolant_Out_Pressure_[kPa]/1 -> Coolant_Out_Pressure_[kPa]/1
  ConvertAnalogTokPa20/1 -> Monitor_Coolant_Out_Pressure_[kPa]/1
  Bus Selector4/1 -> ConvertAnalogTokPa3/1  "<CH1_ANALOG_INPUT_6>"
  Monitor_Crank_Case_Pressure_[kPa]/1 -> Crank_Case_Pressure_[kPa]/1
  ConvertAnalogTokPa5/1 -> Monitor_EGR_In_Pressure_[kPa]/1
  Monitor_EGR_In_Pressure_[kPa]/1 -> EGR_In_Pressure_[kPa]/1
  Bus Selector6/1 -> ConvertAnalogTokPa6/1  "<CH1_ANALOG_INPUT_10>"
  Monitor_Turbine_Front_Pressure_[kPa]/1 -> Turbine_Front_Pressure_[kPa]/1
  ConvertAnalogTokPa6/1 -> Monitor_Turbine_Front_Pressure_[kPa]/1
  Monitor_Turbine_Rear_Pressure_[kPa]/1 -> Turbine_Rear_Pressure_[kPa]/1
  Bus Selector7/1 -> ConvertAnalogTokPa7/1  "<CH1_ANALOG_INPUT_11>"
  Bus Selector8/1 -> ConvertAnalogTokPa9/1  "<CH1_ANALOG_INPUT_14>"
  Monitor_CAC_In_Pressure_[kPa]/1 -> CAC_In_Pressure_[kPa]/1
  Bus Selector2/1 -> ConvertAnalogTokPa8/1  "<CH1_ANALOG_INPUT_12>"
  Monitor_Blowby_Pressure_[kPa]/1 -> Blowby_Pressure_[kPa]/1
  Monitor_Compressor_Out_Pressure_[kPa]/1 -> Compressor_Out_Pressure_[kPa]/1
  Bus Selector9/1 -> ConvertAnalogTokPa10/1  "<CH1_ANALOG_INPUT_15>"
  Bus Selector10/1 -> ConvertAnalogTokPa12/1  "<CH1_ANALOG_INPUT_17>"
  Monitor_CAC_Out_Pressure_[kPa]/1 -> CAC_Out_Pressure_[kPa]/1
  Bus Selector11/1 -> ConvertAnalogTokPa13/1  "<CH1_ANALOG_INPUT_18>"
  Monitor_EGR_Bypass_Out_Pressure_[kPa]/1 -> EGR_Bypass_Out_Pressure_[kPa]/1
  Bus Selector12/1 -> ConvertAnalogTokPa14/1  "<CH1_ANALOG_INPUT_19>"
  ConvertAnalogTokPa14/1 -> Monitor_Intake_Manifold_Pressure_[kPa]/1
  Monitor_Intake_Manifold_Pressure_[kPa]/1 -> Intake_Manifold_Pressure_[kPa]/1
  Monitor_EGR_Cooler_Out_Pressure_[kPa]/1 -> EGR_Cooler_Out_Pressure_[kPa]/1
  Bus Selector13/1 -> ConvertAnalogTokPa15/1  "<CH1_ANALOG_INPUT_21>"
  Bus Selector14/1 -> ConvertAnalogTokPa16/1  "<CH1_ANALOG_INPUT_22>"
  Monitor_Coolant_In_Pressure_[kPa]/1 -> Coolant_In_Pressure_[kPa]/1
  Monitor_EGR_Coolant_In_Pressure_[kPa]/1 -> EGR_Coolant_In_Pressure_[kPa]/1
  ConvertAnalogTokPa17/1 -> Monitor_EGR_Coolant_In_Pressure_[kPa]/1
  Bus Selector15/1 -> ConvertAnalogTokPa17/1  "<CH1_ANALOG_INPUT_23>"
  Bus Selector16/1 -> ConvertAnalogTokPa18/1  "<CH1_ANALOG_INPUT_24>"
  Monitor_EGR_Coolant_Out_Pressure_[kPa]/1 -> EGR_Coolant_Out_Pressure_[kPa]/1
  ConvertAnalogTokPa18/1 -> Monitor_EGR_Coolant_Out_Pressure_[kPa]/1
  ConvertAnalogTokPa19/1 -> Monitor_Block_Intake_Pressure_[kPa]/1
  Bus Selector17/1 -> ConvertAnalogTokPa19/1  "<CH1_ANALOG_INPUT_25>"
  Monitor_Block_Intake_Pressure_[kPa]/1 -> Block_Intake_Pressure_[kPa]/1
  Monitor_Fuel_Pump_In_Pressure_[kPa]/1 -> Fuel_Pump_In_Pressure_[kPa]/1
  ConvertAnalogTokPa1/1 -> Monitor_Fuel_Pump_In_Pressure_[kPa]/1
  Bus Selector18/1 -> ConvertAnalogTokPa1/1  "<CH1_ANALOG_INPUT_3>"
  ConvertAnalogTokPa2/1 -> Monitor_Fuel_Return_Pressure_[kPa]/1
  Monitor_Fuel_Return_Pressure_[kPa]/1 -> Fuel_Return_Pressure_[kPa]/1
  Bus Selector19/1 -> ConvertAnalogTokPa2/1  "<CH1_ANALOG_INPUT_4>"
  ConvertAnalogTokPa/1 -> Monitor_Oil_Refill_Pressure_[kPa]/1
  Monitor_Oil_Refill_Pressure_[kPa]/1 -> Oil_Refill_Pressure_[kPa]/1
  Bus Selector20/1 -> ConvertAnalogTokPa/1  "<CH1_ANALOG_INPUT_2>"
  Analog_Input_Bus/1 -> Bus Selector3/1, Bus Selector17/1, Bus Selector16/1, Bus Selector15/1, Bus Selector14/1, Bus Selector13/1, Bus Selector12/1, Bus Selector11/1, Bus Selector10/1, Bus Selector1/1, Bus Selector9/1, Bus Selector8/1, Bus Selector2/1, Bus Selector7/1, Bus Selector6/1, Bus Selector5/1, Bus Selector/1, Bus Selector4/1, Bus Selector19/1, Bus Selector18/1, Bus Selector20/1
  ConvertAnalogTokPa3/1 -> Monitor_Crank_Case_Pressure_[kPa]/1
  ConvertAnalogTokPa4/1 -> Monitor_Compressor_In_Pressure_[kPa]/1
  Bus Selector5/1 -> ConvertAnalogTokPa5/1  "<CH1_ANALOG_INPUT_8>"
  ConvertAnalogTokPa7/1 -> Monitor_Turbine_Rear_Pressure_[kPa]/1
  ConvertAnalogTokPa8/1 -> Monitor_Blowby_Pressure_[kPa]/1
  ConvertAnalogTokPa9/1 -> Monitor_CAC_In_Pressure_[kPa]/1
  ConvertAnalogTokPa10/1 -> Monitor_Compressor_Out_Pressure_[kPa]/1
  ConvertAnalogTokPa11/1 -> Monitor_Turbine_Out_Pressure_[kPa]/1
  ConvertAnalogTokPa12/1 -> Monitor_CAC_Out_Pressure_[kPa]/1
  ConvertAnalogTokPa13/1 -> Monitor_EGR_Bypass_Out_Pressure_[kPa]/1
  ConvertAnalogTokPa15/1 -> Monitor_EGR_Cooler_Out_Pressure_[kPa]/1
  ConvertAnalogTokPa16/1 -> Monitor_Coolant_In_Pressure_[kPa]/1

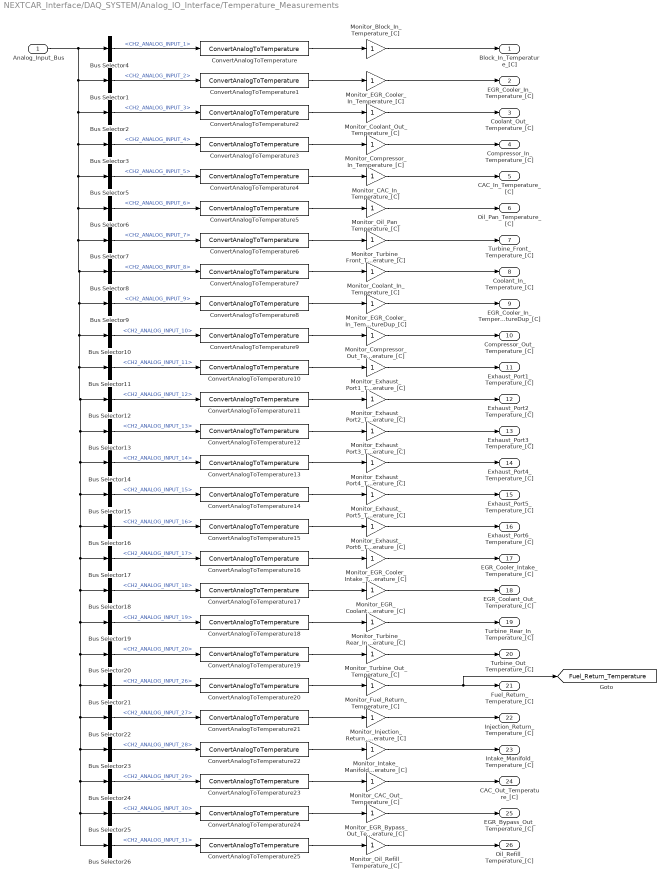
== system NEXTCAR_Interface/DAQ_SYSTEM/Analog_IO_Interface/Temperature_Measurements ==
  Analog_Input_Bus : Inport
  Bus Selector1 : BusSelector  OutputSignals=CH2_ANALOG_INPUTS.CH2_ANALOG_INPUT_2
  Bus Selector10 : BusSelector  OutputSignals=CH2_ANALOG_INPUTS.CH2_ANALOG_INPUT_10
  Bus Selector11 : BusSelector  OutputSignals=CH2_ANALOG_INPUTS.CH2_ANALOG_INPUT_11
  Bus Selector12 : BusSelector  OutputSignals=CH2_ANALOG_INPUTS.CH2_ANALOG_INPUT_12
  Bus Selector13 : BusSelector  OutputSignals=CH2_ANALOG_INPUTS.CH2_ANALOG_INPUT_13
  Bus Selector14 : BusSelector  OutputSignals=CH2_ANALOG_INPUTS.CH2_ANALOG_INPUT_14
  Bus Selector15 : BusSelector  OutputSignals=CH2_ANALOG_INPUTS.CH2_ANALOG_INPUT_15
  Bus Selector16 : BusSelector  OutputSignals=CH2_ANALOG_INPUTS.CH2_ANALOG_INPUT_16
  Bus Selector17 : BusSelector  OutputSignals=CH2_ANALOG_INPUTS.CH2_ANALOG_INPUT_17
  Bus Selector18 : BusSelector  OutputSignals=CH2_ANALOG_INPUTS.CH2_ANALOG_INPUT_18
  Bus Selector19 : BusSelector  OutputSignals=CH2_ANALOG_INPUTS.CH2_ANALOG_INPUT_19
  Bus Selector2 : BusSelector  OutputSignals=CH2_ANALOG_INPUTS.CH2_ANALOG_INPUT_3
  Bus Selector20 : BusSelector  OutputSignals=CH2_ANALOG_INPUTS.CH2_ANALOG_INPUT_20
  Bus Selector21 : BusSelector  OutputSignals=CH2_ANALOG_INPUTS.CH2_ANALOG_INPUT_26
  Bus Selector22 : BusSelector  OutputSignals=CH2_ANALOG_INPUTS.CH2_ANALOG_INPUT_27
  Bus Selector23 : BusSelector  OutputSignals=CH2_ANALOG_INPUTS.CH2_ANALOG_INPUT_28
  Bus Selector24 : BusSelector  OutputSignals=CH2_ANALOG_INPUTS.CH2_ANALOG_INPUT_29
  Bus Selector25 : BusSelector  OutputSignals=CH2_ANALOG_INPUTS.CH2_ANALOG_INPUT_30
  Bus Selector26 : BusSelector  OutputSignals=CH2_ANALOG_INPUTS.CH2_ANALOG_INPUT_31
  Bus Selector3 : BusSelector  OutputSignals=CH2_ANALOG_INPUTS.CH2_ANALOG_INPUT_4
  Bus Selector4 : BusSelector  OutputSignals=CH2_ANALOG_INPUTS.CH2_ANALOG_INPUT_1
  Bus Selector5 : BusSelector  OutputSignals=CH2_ANALOG_INPUTS.CH2_ANALOG_INPUT_5
  Bus Selector6 : BusSelector  OutputSignals=CH2_ANALOG_INPUTS.CH2_ANALOG_INPUT_6
  Bus Selector7 : BusSelector  OutputSignals=CH2_ANALOG_INPUTS.CH2_ANALOG_INPUT_7
  Bus Selector8 : BusSelector  OutputSignals=CH2_ANALOG_INPUTS.CH2_ANALOG_INPUT_8
  Bus Selector9 : BusSelector  OutputSignals=CH2_ANALOG_INPUTS.CH2_ANALOG_INPUT_9
  ConvertAnalogToTemperature{,1..25} (26 alike) : NEXTCAR_Library/ConvertAnalogToTemperature
      settings: SourceProductName=NEXTCAR Library
  Monitor_Block_In_Temperature_[C] : Gain
  Monitor_CAC_In_Temperature_[C] : Gain
  Monitor_CAC_Out_Temperature_[C] : Gain
  Monitor_Compressor_In_Temperature_[C] : Gain
  Monitor_Compressor_Out_Temperature_[C] : Gain
  Monitor_Coolant_In_Temperature_[C] : Gain
  Monitor_Coolant_Out_Temperature_[C] : Gain
  Monitor_EGR_Bypass_Out_Temperature_[C] : Gain
  Monitor_EGR_Coolant_Out_Temperature_[C] : Gain
  Monitor_EGR_Cooler_In_TemperatureDup_[C] : Gain
  Monitor_EGR_Cooler_In_Temperature_[C] : Gain
  Monitor_EGR_Cooler_Intake_Temperature_[C] : Gain
  Monitor_Exhaust_Port1_Temperature_[C] : Gain
  Monitor_Exhaust_Port2_Temperature_[C] : Gain
  Monitor_Exhaust_Port3_Temperature_[C] : Gain
  Monitor_Exhaust_Port4_Temperature_[C] : Gain
  Monitor_Exhaust_Port5_Temperature_[C] : Gain
  Monitor_Exhaust_Port6_Temperature_[C] : Gain
  Monitor_Fuel_Return_Temperature_[C] : Gain
  Monitor_Injection_Return_Temperature_[C] : Gain
  Monitor_Intake_Manifold_Temperature_[C] : Gain
  Monitor_Oil_Pan_Temperature_[C] : Gain
  Monitor_Oil_Refill_Temperature_[C] : Gain
  Monitor_Turbine_Front_Temperature_[C] : Gain
  Monitor_Turbine_Out_Temperature_[C] : Gain
  Monitor_Turbine_Rear_In_Temperature_[C] : Gain
  Block_In_Temperature_[C] : Outport
  EGR_Cooler_In_Temperature_[C] : Outport  Port=2
  Coolant_Out_Temperature_[C] : Outport  Port=3
  Compressor_In_Temperature_[C] : Outport  Port=4
  CAC_In_Temperature_[C] : Outport  Port=5
  Oil_Pan_Temperature_[C] : Outport  Port=6
  Turbine_Front_Temperature_[C] : Outport  Port=7
  Coolant_In_Temperature_[C] : Outport  Port=8
  EGR_Cooler_In_TemperatureDup_[C] : Outport  Port=9
  Compressor_Out_Temperature_[C] : Outport  Port=10
  Exhaust_Port1_Temperature_[C] : Outport  Port=11
  Exhaust_Port2_Temperature_[C] : Outport  Port=12
  Exhaust_Port3_Temperature_[C] : Outport  Port=13
  Exhaust_Port4_Temperature_[C] : Outport  Port=14
  Exhaust_Port5_Temperature_[C] : Outport  Port=15
  Exhaust_Port6_Temperature_[C] : Outport  Port=16
  EGR_Cooler_Intake_Temperature_[C] : Outport  Port=17
  EGR_Coolant_Out_Temperature_[C] : Outport  Port=18
  Turbine_Rear_In_Temperature_[C] : Outport  Port=19
  Turbine_Out_Temperature_[C] : Outport  Port=20
  Fuel_Return_Temperature_[C] : Outport  Port=21
  Injection_Return_Temperature_[C] : Outport  Port=22
  Intake_Manifold_Temperature_[C] : Outport  Port=23
  CAC_Out_Temperature_[C] : Outport  Port=24
  EGR_Bypass_Out_Temperature_[C] : Outport  Port=25
  Oil_Refill_Temperature_[C] : Outport  Port=26
  tag scope: Fuel_Return_Temperature=global
  wires:
  Monitor_Block_In_Temperature_[C]/1 -> Block_In_Temperature_[C]/1
  Bus Selector4/1 -> ConvertAnalogToTemperature/1  "<CH2_ANALOG_INPUT_1>"
  Monitor_EGR_Cooler_In_Temperature_[C]/1 -> EGR_Cooler_In_Temperature_[C]/1
  Bus Selector1/1 -> ConvertAnalogToTemperature1/1  "<CH2_ANALOG_INPUT_2>"
  Bus Selector2/1 -> ConvertAnalogToTemperature2/1  "<CH2_ANALOG_INPUT_3>"
  Monitor_Coolant_Out_Temperature_[C]/1 -> Coolant_Out_Temperature_[C]/1
  Monitor_Compressor_In_Temperature_[C]/1 -> Compressor_In_Temperature_[C]/1
  Bus Selector3/1 -> ConvertAnalogToTemperature3/1  "<CH2_ANALOG_INPUT_4>"
  Bus Selector5/1 -> ConvertAnalogToTemperature4/1  "<CH2_ANALOG_INPUT_5>"
  Monitor_CAC_In_Temperature_[C]/1 -> CAC_In_Temperature_[C]/1
  Monitor_Oil_Pan_Temperature_[C]/1 -> Oil_Pan_Temperature_[C]/1
  Bus Selector6/1 -> ConvertAnalogToTemperature5/1  "<CH2_ANALOG_INPUT_6>"
  Monitor_Turbine_Front_Temperature_[C]/1 -> Turbine_Front_Temperature_[C]/1
  Bus Selector7/1 -> ConvertAnalogToTemperature6/1  "<CH2_ANALOG_INPUT_7>"
  Bus Selector8/1 -> ConvertAnalogToTemperature7/1  "<CH2_ANALOG_INPUT_8>"
  Monitor_Coolant_In_Temperature_[C]/1 -> Coolant_In_Temperature_[C]/1
  Monitor_EGR_Cooler_In_TemperatureDup_[C]/1 -> EGR_Cooler_In_TemperatureDup_[C]/1
  Bus Selector9/1 -> ConvertAnalogToTemperature8/1  "<CH2_ANALOG_INPUT_9>"
  Bus Selector10/1 -> ConvertAnalogToTemperature9/1  "<CH2_ANALOG_INPUT_10>"
  Monitor_Compressor_Out_Temperature_[C]/1 -> Compressor_Out_Temperature_[C]/1
  Bus Selector11/1 -> ConvertAnalogToTemperature10/1  "<CH2_ANALOG_INPUT_11>"
  Monitor_Exhaust_Port1_Temperature_[C]/1 -> Exhaust_Port1_Temperature_[C]/1
  Monitor_Exhaust_Port2_Temperature_[C]/1 -> Exhaust_Port2_Temperature_[C]/1
  Bus Selector12/1 -> ConvertAnalogToTemperature11/1  "<CH2_ANALOG_INPUT_12>"
  Bus Selector13/1 -> ConvertAnalogToTemperature12/1  "<CH2_ANALOG_INPUT_13>"
  Monitor_Exhaust_Port3_Temperature_[C]/1 -> Exhaust_Port3_Temperature_[C]/1
  Monitor_Exhaust_Port4_Temperature_[C]/1 -> Exhaust_Port4_Temperature_[C]/1
  Bus Selector14/1 -> ConvertAnalogToTemperature13/1  "<CH2_ANALOG_INPUT_14>"
  Monitor_Exhaust_Port5_Temperature_[C]/1 -> Exhaust_Port5_Temperature_[C]/1
  Bus Selector15/1 -> ConvertAnalogToTemperature14/1  "<CH2_ANALOG_INPUT_15>"
  Bus Selector16/1 -> ConvertAnalogToTemperature15/1  "<CH2_ANALOG_INPUT_16>"
  Monitor_Exhaust_Port6_Temperature_[C]/1 -> Exhaust_Port6_Temperature_[C]/1
  Monitor_EGR_Cooler_Intake_Temperature_[C]/1 -> EGR_Cooler_Intake_Temperature_[C]/1
  Bus Selector17/1 -> ConvertAnalogToTemperature16/1  "<CH2_ANALOG_INPUT_17>"
  Bus Selector18/1 -> ConvertAnalogToTemperature17/1  "<CH2_ANALOG_INPUT_18>"
  Monitor_EGR_Coolant_Out_Temperature_[C]/1 -> EGR_Coolant_Out_Temperature_[C]/1
  Monitor_Turbine_Rear_In_Temperature_[C]/1 -> Turbine_Rear_In_Temperature_[C]/1
  Bus Selector19/1 -> ConvertAnalogToTemperature18/1  "<CH2_ANALOG_INPUT_19>"
  Monitor_Turbine_Out_Temperature_[C]/1 -> Turbine_Out_Temperature_[C]/1
  Bus Selector20/1 -> ConvertAnalogToTemperature19/1  "<CH2_ANALOG_INPUT_20>"
  ConvertAnalogToTemperature/1 -> Monitor_Block_In_Temperature_[C]/1
  ConvertAnalogToTemperature1/1 -> Monitor_EGR_Cooler_In_Temperature_[C]/1
  ConvertAnalogToTemperature2/1 -> Monitor_Coolant_Out_Temperature_[C]/1
  ConvertAnalogToTemperature3/1 -> Monitor_Compressor_In_Temperature_[C]/1
  ConvertAnalogToTemperature4/1 -> Monitor_CAC_In_Temperature_[C]/1
  ConvertAnalogToTemperature5/1 -> Monitor_Oil_Pan_Temperature_[C]/1
  ConvertAnalogToTemperature6/1 -> Monitor_Turbine_Front_Temperature_[C]/1
  ConvertAnalogToTemperature7/1 -> Monitor_Coolant_In_Temperature_[C]/1
  ConvertAnalogToTemperature8/1 -> Monitor_EGR_Cooler_In_TemperatureDup_[C]/1
  ConvertAnalogToTemperature9/1 -> Monitor_Compressor_Out_Temperature_[C]/1
  ConvertAnalogToTemperature10/1 -> Monitor_Exhaust_Port1_Temperature_[C]/1
  ConvertAnalogToTemperature11/1 -> Monitor_Exhaust_Port2_Temperature_[C]/1
  ConvertAnalogToTemperature12/1 -> Monitor_Exhaust_Port3_Temperature_[C]/1
  ConvertAnalogToTemperature13/1 -> Monitor_Exhaust_Port4_Temperature_[C]/1
  ConvertAnalogToTemperature14/1 -> Monitor_Exhaust_Port5_Temperature_[C]/1
  ConvertAnalogToTemperature15/1 -> Monitor_Exhaust_Port6_Temperature_[C]/1
  ConvertAnalogToTemperature16/1 -> Monitor_EGR_Cooler_Intake_Temperature_[C]/1
  ConvertAnalogToTemperature17/1 -> Monitor_EGR_Coolant_Out_Temperature_[C]/1
  ConvertAnalogToTemperature18/1 -> Monitor_Turbine_Rear_In_Temperature_[C]/1
  ConvertAnalogToTemperature19/1 -> Monitor_Turbine_Out_Temperature_[C]/1
  ConvertAnalogToTemperature20/1 -> Monitor_Fuel_Return_Temperature_[C]/1
  Bus Selector21/1 -> ConvertAnalogToTemperature20/1  "<CH2_ANALOG_INPUT_26>"
  Monitor_Fuel_Return_Temperature_[C]/1 -> [Fuel_Return_Temperature], Fuel_Return_Temperature_[C]/1
  Bus Selector22/1 -> ConvertAnalogToTemperature21/1  "<CH2_ANALOG_INPUT_27>"
  Monitor_Injection_Return_Temperature_[C]/1 -> Injection_Return_Temperature_[C]/1
  ConvertAnalogToTemperature21/1 -> Monitor_Injection_Return_Temperature_[C]/1
  Monitor_Intake_Manifold_Temperature_[C]/1 -> Intake_Manifold_Temperature_[C]/1
  ConvertAnalogToTemperature22/1 -> Monitor_Intake_Manifold_Temperature_[C]/1
  Bus Selector23/1 -> ConvertAnalogToTemperature22/1  "<CH2_ANALOG_INPUT_28>"
  ConvertAnalogToTemperature23/1 -> Monitor_CAC_Out_Temperature_[C]/1
  Monitor_CAC_Out_Temperature_[C]/1 -> CAC_Out_Temperature_[C]/1
  Bus Selector24/1 -> ConvertAnalogToTemperature23/1  "<CH2_ANALOG_INPUT_29>"
  Bus Selector25/1 -> ConvertAnalogToTemperature24/1  "<CH2_ANALOG_INPUT_30>"
  ConvertAnalogToTemperature24/1 -> Monitor_EGR_Bypass_Out_Temperature_[C]/1
  Monitor_EGR_Bypass_Out_Temperature_[C]/1 -> EGR_Bypass_Out_Temperature_[C]/1
  Monitor_Oil_Refill_Temperature_[C]/1 -> Oil_Refill_Temperature_[C]/1
  Analog_Input_Bus/1 -> Bus Selector8/1, Bus Selector26/1, Bus Selector25/1, Bus Selector24/1, Bus Selector23/1, Bus Selector22/1, Bus Selector21/1, Bus Selector20/1, Bus Selector19/1, Bus Selector18/1, Bus Selector17/1, Bus Selector16/1, Bus Selector15/1, Bus Selector14/1, Bus Selector13/1, Bus Selector12/1, Bus Selector11/1, Bus Selector10/1, Bus Selector9/1, Bus Selector7/1, Bus Selector6/1, Bus Selector5/1, Bus Selector3/1, Bus Selector2/1, Bus Selector1/1, Bus Selector4/1
  Bus Selector26/1 -> ConvertAnalogToTemperature25/1  "<CH2_ANALOG_INPUT_31>"
  ConvertAnalogToTemperature25/1 -> Monitor_Oil_Refill_Temperature_[C]/1
